simulink model "PSOmodel"  (R2023a)
settings: Solver=FixedStepAuto  StartTime=0.0  StopTime=19431  FixedStep=1  RelTol=1e-3
undefined symbols (not defined in the file): G, PSO

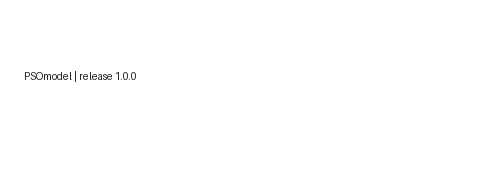
[thumbnail: Simulink's stored preview of the top-level diagram]
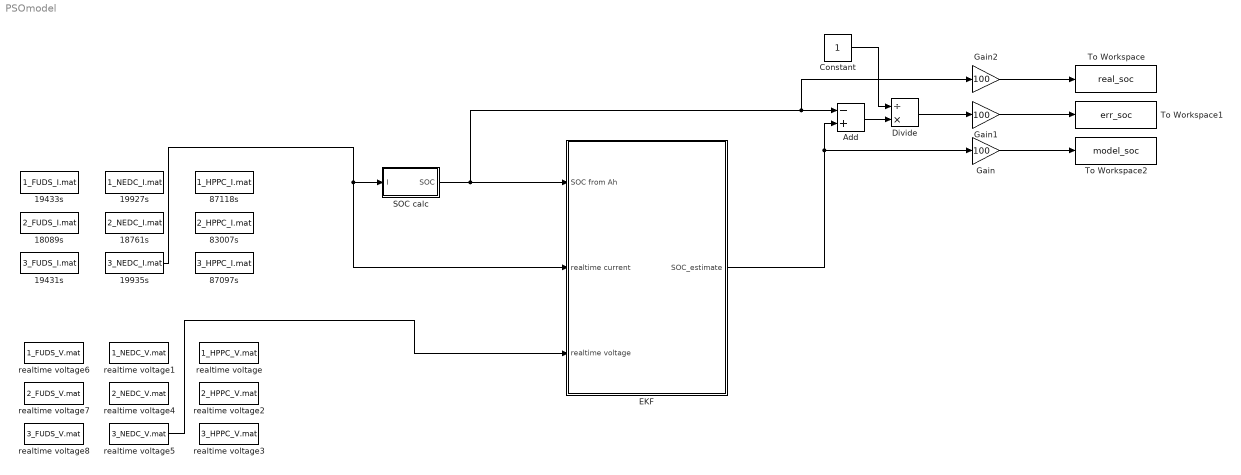
== system PSOmodel ==
  18089s : FromFile  FileName=2_FUDS_I.mat  SampleTime=0
  18761s : FromFile  FileName=2_NEDC_I.mat  SampleTime=0
  19431s : FromFile  FileName=3_FUDS_I.mat  SampleTime=0
  19433s : FromFile  FileName=1_FUDS_I.mat  SampleTime=0
  19927s : FromFile  FileName=1_NEDC_I.mat  SampleTime=0
  19935s : FromFile  FileName=3_NEDC_I.mat  SampleTime=0
  83007s : FromFile  FileName=2_HPPC_I.mat  SampleTime=0
  87097s : FromFile  FileName=3_HPPC_I.mat  SampleTime=0
  87118s : FromFile  FileName=1_HPPC_I.mat  SampleTime=0
  Add : Sum  Inputs=-+
  Constant : Constant
  Divide : Product  Inputs=/*
  EKF : Subsystem
  Gain : Gain  Gain=100
  Gain1 : Gain  Gain=100
  Gain2 : Gain  Gain=100
  SOC calc : Subsystem
  To Workspace : ToWorkspace  VariableName=real_soc  SaveFormat=Timeseries  SampleTime=-1
  To Workspace1 : ToWorkspace  VariableName=err_soc  SaveFormat=Timeseries  SampleTime=-1
  To Workspace2 : ToWorkspace  VariableName=model_soc  SaveFormat=Timeseries  SampleTime=-1
  realtime voltage : FromFile  FileName=1_HPPC_V.mat  SampleTime=0
  realtime voltage1 : FromFile  FileName=1_NEDC_V.mat  SampleTime=0
  realtime voltage2 : FromFile  FileName=2_HPPC_V.mat  SampleTime=0
  realtime voltage3 : FromFile  FileName=3_HPPC_V.mat  SampleTime=0
  realtime voltage4 : FromFile  FileName=2_NEDC_V.mat  SampleTime=0
  realtime voltage5 : FromFile  FileName=3_NEDC_V.mat  SampleTime=0
  realtime voltage6 : FromFile  FileName=1_FUDS_V.mat  SampleTime=0
  realtime voltage7 : FromFile  FileName=2_FUDS_V.mat  SampleTime=0
  realtime voltage8 : FromFile  FileName=3_FUDS_V.mat  SampleTime=0
  wires:
  19935s/1 -> EKF/2(realtime current), SOC calc/1(I)
  EKF/1(SOC_estimate) -> Gain/1, Add/2
  Add/1 -> Divide/2
  realtime voltage5/1 -> EKF/3("realtime voltage ")
  Divide/1 -> Gain1/1
  Gain/1 -> To Workspace2/1
  Constant/1 -> Divide/1
  Gain2/1 -> To Workspace/1
  Gain1/1 -> To Workspace1/1
  SOC calc/1(SOC) -> Gain2/1, Add/1, EKF/1(SOC from Ah)

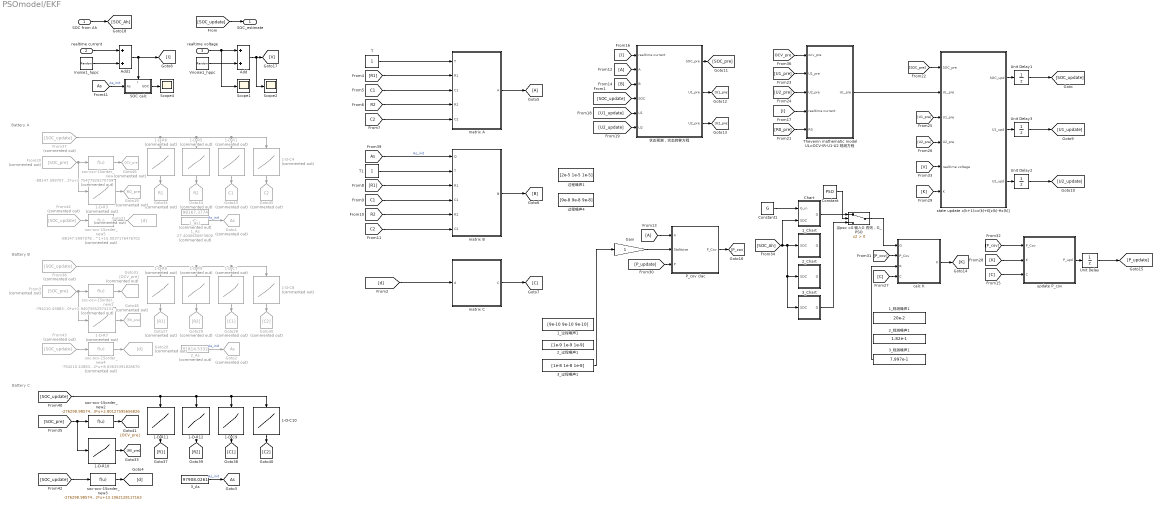
== system PSOmodel/EKF ==
  note: Battery C
  note: Battery B
  note: Battery A
  SOC from Ah : Inport
  realtime current : Inport  Port=2
  "realtime voltage " : Inport  Port=3
  1-D-C10 : Lookup_n-D  NumberOfTableDimensions=1  BreakpointsForDimension1=[2.9109E-07, 0.034704903, 0.080678392, 0.126651918, 0.172626069, 0.218599963, 0.264561539, 0.310535727, 0.35649723, 0.402458916, 0.448432994, 0.494395195, 0.540356772, 0.586318863, 0.632281101, 0.678243265, 0.724205797, 0.770168256, 0.81613042, 0.862092732, 0.908054492, 0.954027467]  Table=[2196.493417, 6254.414395, 10027.09575, 11640.94595, 15150.56735, 14939.39571, 22277.23726, 21788.57636, 21198.25628, 16155.2285, 17423.71863, 20324.46195, 14880.37747, 17370.84513, 17908.76661, 37791.77026, 30450.72328, 20196.6933, 17282.88891, 15011.20802, 15927.09163, 25703.81768]  InternalRulePriority=Speed  RndMeth=Simplest
  1-D-C4 : Lookup_n-D  Commented=on  NumberOfTableDimensions=1  BreakpointsForDimension1=[-1.87350000000000e-16 0.0372369600000000 0.0830859250000000 0.128934580000000 0.174779663000000 0.220625308000000 0.266470959000000 0.312315714000000 0.358160890000000 0.404006225000000 0.449851236000000 0.495695831000000 0.541540865000000 0.587386376000000 0.633231553000000 0.679076361000000 0.724921708000000 0.770765746000000 0.816610252000000 0.862454330000000 0.908300370000000 0.954150372000000]  Table=[128354.582000000 465098.236000000 494756.285300000 743304.727400000 722463.651900000 811208.927300000 406248.240800000 454089.078800000 480121.157400000 703814.335700000 645290.670500000 845206.089900000 863339.383500000 831786.696500000 413452.541700000 382645.914900000 796268.796700000 831394.125000000 798423.035300000 722500.010700000 1812473.80600000 1386271.68100000]  InternalRulePriority=Speed  RndMeth=Simplest
  1-D-C7 : Lookup_n-D  Commented=on  NumberOfTableDimensions=1  BreakpointsForDimension1=[-7.8419E-08, 0.019714291, 0.068728061, 0.117742026, 0.166756071, 0.21576937, 0.264783571, 0.313798204, 0.362812366, 0.411826096, 0.460839905, 0.50985442, 0.55886819, 0.60788247, 0.656896828, 0.705911421, 0.754926406, 0.803941313, 0.852956063, 0.901970617, 0.950985446]  Table=[225214.1434, 187025.2766, 296294.3583, 325129.1549, 382794.7295, 371710.2995, 353976.6676, 381282.3938, 488296.3231, 462238.5316, 712185.7898, 891276.2929, 786232.5864, 455006.0004, 322811.3497, 309379.8901, 321116.448, 741388.8307, 942394.5955, 1060535.922, 1063695.943]  InternalRulePriority=Speed  RndMeth=Simplest
  1-D-C8 : Lookup_n-D  Commented=on  NumberOfTableDimensions=1  BreakpointsForDimension1=[-7.8419E-08, 0.019714291, 0.068728061, 0.117742026, 0.166756071, 0.21576937, 0.264783571, 0.313798204, 0.362812366, 0.411826096, 0.460839905, 0.50985442, 0.55886819, 0.60788247, 0.656896828, 0.705911421, 0.754926406, 0.803941313, 0.852956063, 0.901970617, 0.950985446]  Table=[1671.127633, 1673.968389, 4565.243665, 6209.535618, 11242.6131, 9787.657058, 11449.06044, 14014.79555, 15699.36024, 13663.69917, 14717.09328, 14685.37445, 16462.66037, 11898.52641, 12704.67604, 16178.70649, 18177.54925, 20734.64693, 17610.56739, 15941.06135, 15784.62672]  InternalRulePriority=Speed  RndMeth=Simplest
  1-D-C9 : Lookup_n-D  NumberOfTableDimensions=1  BreakpointsForDimension1=[2.9109E-07, 0.034704903, 0.080678392, 0.126651918, 0.172626069, 0.218599963, 0.264561539, 0.310535727, 0.35649723, 0.402458916, 0.448432994, 0.494395195, 0.540356772, 0.586318863, 0.632281101, 0.678243265, 0.724205797, 0.770168256, 0.81613042, 0.862092732, 0.908054492, 0.954027467]  Table=[148211.7874, 379943.691, 507178.8648, 540877.9099, 565031.5977, 599113.5276, 468851.5567, 439228.3613, 564632.19, 525250.0917, 713932.6032, 938377.816, 623343.6413, 597265.7355, 374444.1491, 318686.1875, 638311.9656, 790877.9592, 883896.1639, 825362.4483, 795349.2136, 1510862.771]  InternalRulePriority=Speed  RndMeth=Simplest
  1-D-R1 : Lookup_n-D  Commented=on  NumberOfTableDimensions=1  BreakpointsForDimension1=[-1.87350000000000e-16 0.0372369600000000 0.0830859250000000 0.128934580000000 0.174779663000000 0.220625308000000 0.266470959000000 0.312315714000000 0.358160890000000 0.404006225000000 0.449851236000000 0.495695831000000 0.541540865000000 0.587386376000000 0.633231553000000 0.679076361000000 0.724921708000000 0.770765746000000 0.816610252000000 0.862454330000000 0.908300370000000 0.954150372000000]  Table=[0.00810316000000000 0.00251698500000000 0.00186214400000000 0.00178860800000000 0.00152974100000000 0.00147679700000000 0.00190128400000000 0.00201018500000000 0.00174515000000000 0.00143752800000000 0.00133514600000000 0.00126586900000000 0.00125399700000000 0.00138251100000000 0.00279094200000000 0.00218289100000000 0.00138689300000000 0.00122421400000000 0.00113694900000000 0.00107976200000000 0.000788270000000000 0.000893057000000000]  InternalRulePriority=Speed  RndMeth=Simplest
  1-D-R10 : Lookup_n-D  NumberOfTableDimensions=1  BreakpointsForDimension1=[2.9109E-07, 0.034704903, 0.080678392, 0.126651918, 0.172626069, 0.218599963, 0.264561539, 0.310535727, 0.35649723, 0.402458916, 0.448432994, 0.494395195, 0.540356772, 0.586318863, 0.632281101, 0.678243265, 0.724205797, 0.770168256, 0.81613042, 0.862092732, 0.908054492, 0.954027467]  Table=[0.002528647, 0.001936736, 0.001933092, 0.002009272, 0.001857034, 0.001932965, 0.001937093, 0.001860779, 0.001865146, 0.001940916, 0.001785007, 0.001860795, 0.001784893, 0.001792897, 0.001860957, 0.001860919, 0.001788901, 0.0017849, 0.001708766, 0.001708843, 0.001636824, 0.001636826]  InternalRulePriority=Speed  RndMeth=Simplest
  1-D-R11 : Lookup_n-D  NumberOfTableDimensions=1  BreakpointsForDimension1=[2.9109E-07, 0.034704903, 0.080678392, 0.126651918, 0.172626069, 0.218599963, 0.264561539, 0.310535727, 0.35649723, 0.402458916, 0.448432994, 0.494395195, 0.540356772, 0.586318863, 0.632281101, 0.678243265, 0.724205797, 0.770168256, 0.81613042, 0.862092732, 0.908054492, 0.954027467]  Table=[0.007426917, 0.002725754, 0.002056684, 0.002051955, 0.001788462, 0.001933155, 0.002069724, 0.00225684, 0.001884435, 0.0016594, 0.001488249, 0.001395496, 0.001419538, 0.001566898, 0.002844649, 0.002781912, 0.001682693, 0.00138196, 0.001233272, 0.001177427, 0.001101257, 0.000924041]  InternalRulePriority=Speed  RndMeth=Simplest
  1-D-R12 : Lookup_n-D  NumberOfTableDimensions=1  BreakpointsForDimension1=[2.9109E-07, 0.034704903, 0.080678392, 0.126651918, 0.172626069, 0.218599963, 0.264561539, 0.310535727, 0.35649723, 0.402458916, 0.448432994, 0.494395195, 0.540356772, 0.586318863, 0.632281101, 0.678243265, 0.724205797, 0.770168256, 0.81613042, 0.862092732, 0.908054492, 0.954027467]  Table=[0.012678994, 0.006218342, 0.004585322, 0.003481865, 0.003212414, 0.002922909, 0.002535113, 0.002663285, 0.002728817, 0.002644002, 0.002455207, 0.0022745, 0.002186381, 0.002057863, 0.001998786, 0.002105164, 0.002862673, 0.002808045, 0.002531815, 0.002274687, 0.00198128, 0.001756841]  InternalRulePriority=Speed  RndMeth=Simplest
  1-D-R3 : Lookup_n-D  Commented=on  NumberOfTableDimensions=1  BreakpointsForDimension1=[-1.87350000000000e-16 0.0372369600000000 0.0830859250000000 0.128934580000000 0.174779663000000 0.220625308000000 0.266470959000000 0.312315714000000 0.358160890000000 0.404006225000000 0.449851236000000 0.495695831000000 0.541540865000000 0.587386376000000 0.633231553000000 0.679076361000000 0.724921708000000 0.770765746000000 0.816610252000000 0.862454330000000 0.908300370000000 0.954150372000000]  Table=[0.00237719800000000 0.00193720900000000 0.00163261400000000 0.00164061700000000 0.00163282300000000 0.00148875000000000 0.00148875000000000 0.00164061700000000 0.00164082700000000 0.00148892900000000 0.00148912000000000 0.00148875000000000 0.00148875000000000 0.00148875000000000 0.00148875000000000 0.00148856000000000 0.00148892900000000 0.00134450600000000 0.00134467800000000 0.00148856000000000 0.00164082700000000 0.00148856000000000]  InternalRulePriority=Speed  RndMeth=Simplest
  1-D-R5 : Lookup_n-D  Commented=on  NumberOfTableDimensions=1  BreakpointsForDimension1=[-1.87350000000000e-16 0.0372369600000000 0.0830859250000000 0.128934580000000 0.174779663000000 0.220625308000000 0.266470959000000 0.312315714000000 0.358160890000000 0.404006225000000 0.449851236000000 0.495695831000000 0.541540865000000 0.587386376000000 0.633231553000000 0.679076361000000 0.724921708000000 0.770765746000000 0.816610252000000 0.862454330000000 0.908300370000000 0.954150372000000]  Table=[0.00810316000000000 0.00251698500000000 0.00186214400000000 0.00178860800000000 0.00152974100000000 0.00147679700000000 0.00190128400000000 0.00201018500000000 0.00174515000000000 0.00143752800000000 0.00133514600000000 0.00126586900000000 0.00125399700000000 0.00138251100000000 0.00279094200000000 0.00218289100000000 0.00138689300000000 0.00122421400000000 0.00113694900000000 0.00107976200000000 0.000788270000000000 0.000893057000000000]  InternalRulePriority=Speed  RndMeth=Simplest
  1-D-R6 : Lookup_n-D  Commented=on  NumberOfTableDimensions=1  BreakpointsForDimension1=[-1.87350000000000e-16 0.0372369600000000 0.0830859250000000 0.128934580000000 0.174779663000000 0.220625308000000 0.266470959000000 0.312315714000000 0.358160890000000 0.404006225000000 0.449851236000000 0.495695831000000 0.541540865000000 0.587386376000000 0.633231553000000 0.679076361000000 0.724921708000000 0.770765746000000 0.816610252000000 0.862454330000000 0.908300370000000 0.954150372000000]  Table=[0.00853642300000000 0.00464516200000000 0.00372978500000000 0.00280459900000000 0.00271064400000000 0.00238071300000000 0.00215293400000000 0.00228803900000000 0.00239974300000000 0.00228676500000000 0.00209879800000000 0.00194772300000000 0.00181591800000000 0.00170293300000000 0.00173486000000000 0.00212977600000000 0.00261638200000000 0.00242766200000000 0.00219563000000000 0.00194553200000000 0.00171752800000000 0.00157829700000000]  InternalRulePriority=Speed  RndMeth=Simplest
  1-D-R7 : Lookup_n-D  Commented=on  NumberOfTableDimensions=1  BreakpointsForDimension1=[-7.8419E-08, 0.019714291, 0.068728061, 0.117742026, 0.166756071, 0.21576937, 0.264783571, 0.313798204, 0.362812366, 0.411826096, 0.460839905, 0.50985442, 0.55886819, 0.60788247, 0.656896828, 0.705911421, 0.754926406, 0.803941313, 0.852956063, 0.901970617, 0.950985446]  Table=[0.005142418, 0.004920407, 0.004844512, 0.004848168, 0.00477236, 0.004844207, 0.004916611, 0.004768351, 0.004768354, 0.004767743, 0.004920582, 0.00484046, 0.004695644, 0.004619808, 0.004547664, 0.004543704, 0.004467293, 0.004547664, 0.004547368, 0.004399462, 0.004246964]  InternalRulePriority=Speed  RndMeth=Simplest
  1-D-R8 : Lookup_n-D  Commented=on  NumberOfTableDimensions=1  BreakpointsForDimension1=[-7.8419E-08, 0.019714291, 0.068728061, 0.117742026, 0.166756071, 0.21576937, 0.264783571, 0.313798204, 0.362812366, 0.411826096, 0.460839905, 0.50985442, 0.55886819, 0.60788247, 0.656896828, 0.705911421, 0.754926406, 0.803941313, 0.852956063, 0.901970617, 0.950985446]  Table=[0.00461437, 0.004542772, 0.002927848, 0.002489007, 0.00261231, 0.002854022, 0.002839665, 0.002705643, 0.002322517, 0.001930102, 0.001569536, 0.001434529, 0.001559029, 0.002338951, 0.003742684, 0.00311492, 0.00238201, 0.001540864, 0.001263662, 0.001122294, 0.001006783]  InternalRulePriority=Speed  RndMeth=Simplest
  1-D-R9 : Lookup_n-D  Commented=on  NumberOfTableDimensions=1  BreakpointsForDimension1=[-7.8419E-08, 0.019714291, 0.068728061, 0.117742026, 0.166756071, 0.21576937, 0.264783571, 0.313798204, 0.362812366, 0.411826096, 0.460839905, 0.50985442, 0.55886819, 0.60788247, 0.656896828, 0.705911421, 0.754926406, 0.803941313, 0.852956063, 0.901970617, 0.950985446]  Table=[0.022805443, 0.021704309, 0.009347226, 0.005943316, 0.004810936, 0.004550218, 0.004093036, 0.003809411, 0.003763955, 0.003626777, 0.003515244, 0.003368593, 0.002718876, 0.003041587, 0.003017746, 0.002947958, 0.003081328, 0.00338066, 0.003232809, 0.003004131, 0.002690434]  InternalRulePriority=Speed  RndMeth=Simplest
  1_As : Constant  Commented=on  Value=27.40406506*3600
  1_As1 : Constant  Commented=on  Value=98167.3774
  1_Chart : Stateflow chart  TreatAsAtomicUnit=on
  1_观测噪声1 : Constant  Value=20e-2
  1_过程噪声1 : Constant  Value=[9e-10 9e-10 9e-10]
  2_As : Constant  Commented=on  Value=91814.5332
  2_Chart : Stateflow chart  TreatAsAtomicUnit=on
  2_观测噪声1 : Constant  Value=1.82e-1
  2_过程噪声1 : Constant  Value=[1e-9 1e-9 1e-9]
  3_As : Constant  Value=97908.0261
  3_Chart : Stateflow chart  TreatAsAtomicUnit=on
  3_观测噪声1 : Constant  Value=7.997e-1  VectorParams1D=off
  3_过程噪声1 : Constant  Value=[1e-8 1e-8 1e-8]
  Add : Sum
  Add1 : Sum
  Chart : Stateflow chart  TreatAsAtomicUnit=on
      settings: PortSchema="{\"entries\":[{\"content\":{\"sides\":[{\"content\":{\"connectorIds\":[\"In2\",\"In1\"]},\"type\":\"ConnectorPlacement.EquallySpacedRectSide\",\"uuid\":\"e7012a5c-4e88-428d-83d6-0abb774271f4\"},{\"content\":{\"connectorIds\":[\"Out1\"],\"side\":\"RIGHT\"},\"type\":\"ConnectorPlacement.EquallySpacedRectSide\",\"uuid\":\"a64351c2-cb69-49cc-89e3-a743088e35f9\"},{\"content\":{\"side\":\"TOP\"},\"type\":\"ConnectorPlacement.EquallySpacedRectSide\",\"uuid\":\"04fad1cd-d4dd-41b0-a559-7d397359cb8e\"}]},\"type\":\"ConnectorPlacement.EquallySpacedConnector\",\"uuid\":\"62b6021a-e1f5-4386-ac4f-7a5c61b690a4\"}],\"packageUris\":[\"http://schema.mathworks.com/mf0/Connector/R2020b\"],\"version\":\"1.0\"}"
  Constant : Constant  Value=PSO
  Constant1 : Constant  Value=G
  From12 : From
  From13 : From
  From20 : From  Commented=on  GotoTag=SOC_pre
  From3 : From  Commented=on  GotoTag=SOC_pre
  From{37..38,43..44} (4 alike) : From  Commented=on  GotoTag=SOC_update
  Gain : Gain
  Goto1 : Goto  Commented=on  GotoTag=As  TagVisibility=global
  Goto19 : Goto  Commented=on  GotoTag=R0_pre  TagVisibility=global
  Goto2 : Goto  Commented=on  GotoTag=As  TagVisibility=global
  Goto20 : Goto  Commented=on  GotoTag=d
  Goto21 : Goto  Commented=on  GotoTag=d
  Goto27 : Goto  Commented=on  GotoTag=R1
  Goto28 : Goto  Commented=on  GotoTag=C1
  Goto29 : Goto  Commented=on  GotoTag=R2
  Goto30 : Goto  Commented=on  GotoTag=C2
  Goto31 : Goto  Commented=on  GotoTag=OCV_pre
  Goto34 : Goto  Commented=on  GotoTag=R1  TagVisibility=global
  Goto43 : Goto  Commented=on  GotoTag=C1  TagVisibility=global
  Goto44 : Goto  Commented=on  GotoTag=R2  TagVisibility=global
  Goto45 : Goto  Commented=on  GotoTag=C2  TagVisibility=global
  Goto46 : Goto  Commented=on  GotoTag=OCV_pre  TagVisibility=global
  Goto48 : Goto  Commented=on  GotoTag=R0_pre
  Goto5 : Goto
  Inoise1_hppc : RandomNumber  Mean=0.01  Variance=1e-7  SampleTime=0
  P_cov clac : MATLAB Function  TreatAsAtomicUnit=on
  SOC calc : Subsystem
      settings: PortSchema="{\"entries\":[{\"content\":{\"sides\":[{\"content\":{\"connectorIds\":[\"In1\"]},\"type\":\"ConnectorPlacement.EquallySpacedRectSide\",\"uuid\":\"9a15624f-070f-46ab-b122-3cccf513f6e5\"},{\"content\":{\"connectorIds\":[\"Out1\"],\"side\":\"RIGHT\"},\"type\":\"ConnectorPlacement.EquallySpacedRectSide\",\"uuid\":\"7075dd8f-f637-4b75-9ab6-2a45eadbfae6\"},{\"content\":{\"connectorIds\":[\"In2\"],\"side\":\"TOP\"},\"type\":\"ConnectorPlacement.EquallySpacedRectSide\",\"uuid\":\"a2ff706a-1abd-4808-a923-af34f3449a3c\"}]},\"type\":\"ConnectorPlacement.EquallySpacedConnector\",\"uuid\":\"893fac7f-2ce4-44cf-9782-68cb5d4c65ac\"}],\"packageUris\":[\"http://schema.mathworks.com/mf0/Connector/R2020b\"],\"version\":\"1.0\"}"
  Scope1 : Scope
  Scope2 : Scope
  Scope4 : Scope
  T : Constant
  T1 : Constant
  Thevenin mathematic model UL=OCV-IR-U1-U2 观测方程 : Subsystem  TreatAsAtomicUnit=on
  Unit Delay : UnitDelay  InitialCondition=[0.01,0,0,0,0.01,0,0,0,0.01]  SampleTime=-1  HasFrameUpgradeWarning=on
  Unit Delay1 : UnitDelay  InitialCondition=0.95  HasFrameUpgradeWarning=on
  Unit Delay2 : UnitDelay  InitialCondition=0.5  HasFrameUpgradeWarning=on
  Unit Delay3 : UnitDelay  InitialCondition=0.5  HasFrameUpgradeWarning=on
  Vnoise1_hppc : RandomNumber  Mean=0.001  Variance=1e-9  SampleTime=0
  calc K : MATLAB Function  TreatAsAtomicUnit=on
  matrix A : Subsystem  TreatAsAtomicUnit=on
  matrix B : Subsystem  TreatAsAtomicUnit=on
  matrix C : Subsystem  TreatAsAtomicUnit=on
  soc-ocv-15order_new : Fcn  Commented=on  Expr=-88147.5997078394*u^15+790326.983827153*u^14-3193562.76566965*u^13+7683743.41545882*u^12-12242299.9696135*u^11+13582405.847664*u^10-10735891.8510933*u^9+6074345.19664904*u^8-2430691.37715694*u^7+664003.897026294*u^6-113520.233149201*u^5+8942.36593610576*u^4+511.723044470873*u^3-179.974721169225*u^2+15.0037176476702*u+2.75477929270709
  soc-ocv-15order_new1 : Fcn  Commented=on  Expr=-794210.438834610*u^15+5987745.61568300*u^14-20439836.7898101*u^13+41772168.8258101*u^12-56921777.5690841*u^11+54490938.0492044*u^10-37586563.2858994*u^9+18834958.2927790*u^8-6814558.32935900*u^7+1740625.65248685*u^6-299189.844437199*u^5+31109.3414812153*u^4-1360.69378520401*u^3-57.0272510664786*u^2+8.63635391828670*u+2.94075652974131
  soc-ocv-15order_new2 : Fcn  Expr=-276298.985749310*u^15+2079100.19510310*u^14-7146107.09932892*u^13+14857923.9617195*u^12-20833240.2231729*u^11+20756759.1140984*u^10-15054210.4175051*u^9+7991543.21304879*u^8-3070959.05248522*u^7+827625.466792177*u^6-145769.880033493*u^5+13780.6338711194*u^4-19.7560716602156*u^3-139.705484335419*u^2+13.1062128117163*u+2.80127595656826
  soc-ocv-15order_new3 : Fcn  Expr=-276298.985749310*15*u^14+2079100.19510310*14*u^13-7146107.09932892*13*u^12+14857923.9617195*12*u^11-20833240.2231729*11*u^10+20756759.1140984*10*u^9-15054210.4175051*9*u^8+7991543.21304879*8*u^7-3070959.05248522*7*u^6+827625.466792177*6*u^5-145769.880033493*5*u^4+13780.6338711194*4*u^3-19.7560716602156*3*u^2-139.705484335419*2*u+13.1062128117163
  soc-ocv-15order_new4 : Fcn  Commented=on  Expr=-794210.438834610*15*u^14+5987745.61568300*14*u^13-20439836.7898101*13*u^12+41772168.8258101*12*u^11-56921777.5690841*11*u^10+54490938.0492044*10*u^9-37586563.2858994*9*u^8+18834958.2927790*8*u^7-6814558.32935900*7*u^6+1740625.65248685*6*u^5-299189.844437199*5*u^4+31109.3414812153*4*u^3-1360.69378520401*3*u^2-57.0272510664786*2*u+8.63635391828670
  soc-ocv-15order_new5 : Fcn  Commented=on  Expr=-88147.5997078394*15*u^14+790326.983827153*14*u^13-3193562.76566965*13*u^12+7683743.41545882*12*u^11-12242299.9696135*11*u^10+13582405.847664*10*u^9-10735891.8510933*9*u^8+6074345.19664904*8*u^7-2430691.37715694*7*u^6+664003.897026294*6*u^5-113520.233149201*5*u^4+8942.36593610576*4*u^3+511.723044470873*3*u^2-179.974721169225*2*u^1+15.0037176476702
  state update x(k+1)=x(k)+K[z(k)-Hx(k)] : Subsystem
  update P_cov : MATLAB Function  TreatAsAtomicUnit=on
  当pso >0 输入G 否则，G_PSO : Switch  Criteria=u2 > Threshold  SaturateOnIntegerOverflow=off  InputSameDT=off
  状态预测，状态转移方程 : Subsystem
  过程噪声1 : Constant  Value=[2e-5 1e-5 1e-5]
  过程噪声4 : Constant  Value=[9e-8 9e-8 9e-8]
  SOC_estimate : Outport
  tag scope: As=global
  wires:
  [As] -> matrix B/1(Q)  "As_init"
  [C] -> update P_cov/3(C)
  [U2_pre] -> Thevenin mathematic model UL=OCV-IR-U1-U2 观测方程/3(U2_pre)
  [OCV_pre] -> Thevenin mathematic model UL=OCV-IR-U1-U2 观测方程/1(ocv_pre)
  [U1_pre] -> Thevenin mathematic model UL=OCV-IR-U1-U2 观测方程/2(U1_pre)
  state update x(k+1)=x(k)+K[z(k)-Hx(k)]/2(U1_upd) -> Unit Delay3/1
  state update x(k+1)=x(k)+K[z(k)-Hx(k)]/3(U2_upd) -> Unit Delay2/1
  T/1 -> matrix A/1(T)
  state update x(k+1)=x(k)+K[z(k)-Hx(k)]/1(SOC_upd) -> Unit Delay1/1
  Thevenin mathematic model UL=OCV-IR-U1-U2 观测方程/1(UL_pre) -> state update x(k+1)=x(k)+K[z(k)-Hx(k)]/2(UL_pre)
  update P_cov/1(P_upd) -> Unit Delay/1
  Gain/1 -> P_cov clac/2(StaNoise)
  3_Chart/1(G) -> 当pso >0 输入G 否则，G_PSO/3
  [SOC_update] -> SOC_estimate/1
  T1/1 -> matrix B/2(T)
  [SOC_update] -> 状态预测，状态转移方程/4(SOC)
  [d] -> matrix C/1(d)
  [R1] -> matrix A/2(R1)
  [C1] -> matrix A/3(C1)
  [R2] -> matrix A/4(R2)
  [C2] -> matrix A/5(C2)
  [R1] -> matrix B/3(R1)
  [C1] -> matrix B/4(C1)
  [R2] -> matrix B/5(R2)
  [C2] -> matrix B/6(C2)
  matrix A/1(A) -> Goto5/1
  matrix B/1(B) -> [B]
  From12/1 -> 状态预测，状态转移方程/2(A)
  From13/1 -> P_cov clac/1(A)
  [B] -> 状态预测，状态转移方程/3(B)
  matrix C/1(C) -> [C]
  realtime current/1 -> Add1/1
  [I] -> 状态预测，状态转移方程/1(realtime current)
  [I] -> Thevenin mathematic model UL=OCV-IR-U1-U2 观测方程/4(realtime current)
  Unit Delay3/1 -> [U1_update]
  Unit Delay2/1 -> [U2_update]
  [U1_update] -> 状态预测，状态转移方程/5(U1)
  [U2_update] -> 状态预测，状态转移方程/6(U2)
  [SOC_pre] -> state update x(k+1)=x(k)+K[z(k)-Hx(k)]/1(SOC_pre)
  状态预测，状态转移方程/2(U1_pre) -> [U1_pre]
  状态预测，状态转移方程/3(U2_pre) -> [U2_pre]
  [U1_pre] -> state update x(k+1)=x(k)+K[z(k)-Hx(k)]/3(U1_pre)
  [U2_pre] -> state update x(k+1)=x(k)+K[z(k)-Hx(k)]/4(U2_pre)
  [C] -> calc K/4(C)
  calc K/1(K) -> [K]
  [K] -> update P_cov/2(K)
  [K] -> state update x(k+1)=x(k)+K[z(k)-Hx(k)]/6(K)
  Unit Delay/1 -> [P_update]
  [P_update] -> P_cov clac/3(P)
  P_cov clac/1(P_Cov) -> [P_cov]
  [P_cov] -> calc K/2(P_Cov)
  [P_cov] -> update P_cov/1(P_Cov)
  [V] -> state update x(k+1)=x(k)+K[z(k)-Hx(k)]/5(realtime voltage)
  SOC from Ah/1 -> [SOC_Ah]
  [SOC_Ah] -> Chart/1(SOC), 3_Chart/1(SOC), 2_Chart/1(SOC), 1_Chart/1(SOC)
  [R0_pre] -> Thevenin mathematic model UL=OCV-IR-U1-U2 观测方程/5(R0)
  Inoise1_hppc/1 -> Add1/2
  Add1/1 -> SOC calc/2(I), [I]
  Vnoise1_hppc/1 -> Add/2
  Add/1 -> Scope2/1, [V]
  "realtime voltage "/1 -> Scope1/1, Add/1
  状态预测，状态转移方程/1(SOC_pre) -> [SOC_pre]
  SOC calc/1(SOC) -> Scope4/1
  Unit Delay1/1 -> [SOC_update]
  soc-ocv-15order_new2/1 -> [OCV_pre]
  1-D-C4/1 -> Goto45/1
  1-D-R12/1 -> [R2]
  1-D-R11/1 -> [R1]
  From37/1 -> 1-D-R6/1, 1-D-R5/1, 1-D-C4/1, 1-D-R1/1
  1-D-C10/1 -> [C2]
  1-D-R9/1 -> Goto29/1
  1-D-R10/1 -> [R0_pre]
  From38/1 -> 1-D-C8/1, 1-D-C7/1, 1-D-R9/1, 1-D-R8/1
  [SOC_update] -> 1-D-C10/1, 1-D-C9/1, 1-D-R12/1, 1-D-R11/1
  1-D-R8/1 -> Goto27/1
  1-D-R5/1 -> Goto44/1
  1-D-R3/1 -> Goto19/1
  1-D-R7/1 -> Goto48/1
  soc-ocv-15order_new1/1 -> Goto31/1
  1-D-C8/1 -> Goto30/1
  1-D-C7/1 -> Goto28/1
  1-D-R1/1 -> Goto43/1
  1-D-R6/1 -> Goto34/1
  soc-ocv-15order_new/1 -> Goto46/1
  1-D-C9/1 -> [C1]
  From20/1 -> 1-D-R3/1, soc-ocv-15order_new/1
  From3/1 -> soc-ocv-15order_new1/1, 1-D-R7/1
  [SOC_pre] -> 1-D-R10/1, soc-ocv-15order_new2/1
  [As] -> SOC calc/1(As)  "As_init"
  1_As/1 -> Goto1/1  "As_init"
  3_As/1 -> [As]  "As_init"
  2_As/1 -> Goto2/1  "As_init"
  [SOC_update] -> soc-ocv-15order_new3/1
  soc-ocv-15order_new3/1 -> [d]
  soc-ocv-15order_new4/1 -> Goto20/1
  From43/1 -> soc-ocv-15order_new4/1
  soc-ocv-15order_new5/1 -> Goto21/1
  From44/1 -> soc-ocv-15order_new5/1
  3_过程噪声1/1 -> Gain/1
  3_观测噪声1/1 -> calc K/3(R)
  当pso >0 输入G 否则，G_PSO/1 -> calc K/1(G)
  Constant/1 -> 当pso >0 输入G 否则，G_PSO/2
  Chart/1(G) -> 当pso >0 输入G 否则，G_PSO/1
  Constant1/1 -> Chart/2(G_in)

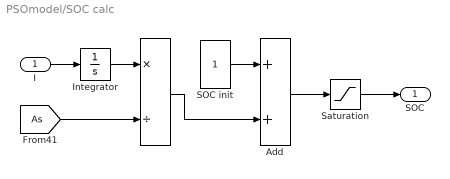
== system PSOmodel/SOC calc ==
  I : Inport
  "     " : Product  Inputs=*/
  Add : Sum
  Integrator : Integrator
  SOC init : Constant
  Saturation : Saturate  UpperLimit=1  LowerLimit=0
  SOC : Outport  VectorParamsAs1DForOutWhenUnconnected=off
  wires:
  [As] -> "     "/2
  Saturation/1 -> SOC/1
  SOC init/1 -> Add/1
  I/1 -> Integrator/1
  Integrator/1 -> "     "/1
  "     "/1 -> Add/2
  Add/1 -> Saturation/1

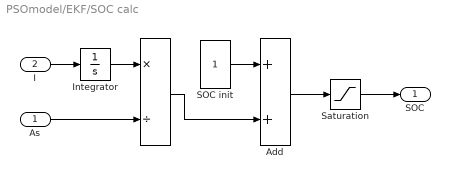
== system PSOmodel/EKF/SOC calc ==
  As : Inport
  I : Inport  Port=2
  "     " : Product  Inputs=*/
  Add : Sum
  Integrator : Integrator
  SOC init : Constant
  Saturation : Saturate  UpperLimit=1  LowerLimit=0
  SOC : Outport  VectorParamsAs1DForOutWhenUnconnected=off
  wires:
  As/1 -> "     "/2
  Saturation/1 -> SOC/1
  SOC init/1 -> Add/1
  I/1 -> Integrator/1
  Integrator/1 -> "     "/1
  "     "/1 -> Add/2
  Add/1 -> Saturation/1

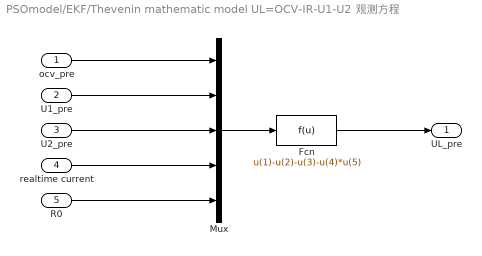
== system PSOmodel/EKF/Thevenin mathematic model UL=OCV-IR-U1-U2 观测方程 ==
  ocv_pre : Inport
  U1_pre : Inport  Port=2
  U2_pre : Inport  Port=3
  realtime current : Inport  Port=4
  R0 : Inport  Port=5
  Fcn : Fcn  Expr=u(1)-u(2)-u(3)-u(4)*u(5)
  Mux : Mux  Inputs=5
  UL_pre : Outport  VectorParamsAs1DForOutWhenUnconnected=off
  wires:
  Mux/1 -> Fcn/1
  ocv_pre/1 -> Mux/1
  U1_pre/1 -> Mux/2
  Fcn/1 -> UL_pre/1
  realtime current/1 -> Mux/4
  R0/1 -> Mux/5
  U2_pre/1 -> Mux/3

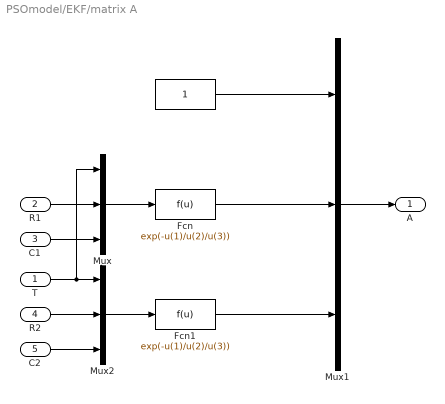
== system PSOmodel/EKF/matrix A ==
  T : Inport
  R1 : Inport  Port=2
  C1 : Inport  Port=3
  R2 : Inport  Port=4
  C2 : Inport  Port=5
  " " : Constant
  Fcn : Fcn  Expr=exp(-u(1)/u(2)/u(3))
  Fcn1 : Fcn  Expr=exp(-u(1)/u(2)/u(3))
  Mux : Mux  Inputs=3
  Mux1 : Mux  Inputs=3
  Mux2 : Mux  Inputs=3
  A : Outport  VectorParamsAs1DForOutWhenUnconnected=off
  wires:
  R1/1 -> Mux/2
  Fcn/1 -> Mux1/2
  T/1 -> Mux/1, Mux2/1
  C1/1 -> Mux/3
  Mux/1 -> Fcn/1
  " "/1 -> Mux1/1
  Mux1/1 -> A/1
  R2/1 -> Mux2/2
  C2/1 -> Mux2/3
  Mux2/1 -> Fcn1/1
  Fcn1/1 -> Mux1/3

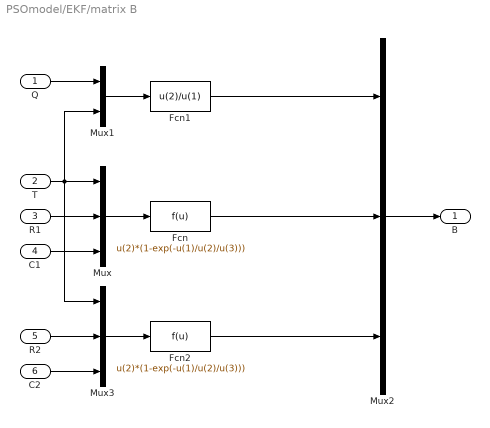
== system PSOmodel/EKF/matrix B ==
  Q : Inport
  T : Inport  Port=2
  R1 : Inport  Port=3
  C1 : Inport  Port=4
  R2 : Inport  Port=5
  C2 : Inport  Port=6
  Fcn : Fcn  Expr=u(2)*(1-exp(-u(1)/u(2)/u(3)))
  Fcn1 : Fcn  Expr=u(2)/u(1)
  Fcn2 : Fcn  Expr=u(2)*(1-exp(-u(1)/u(2)/u(3)))
  Mux : Mux  Inputs=3
  Mux1 : Mux  Inputs=2
  Mux2 : Mux  Inputs=3
  Mux3 : Mux  Inputs=3
  B : Outport  VectorParamsAs1DForOutWhenUnconnected=off
  wires:
  R1/1 -> Mux/2
  T/1 -> Mux3/1, Mux1/2, Mux/1
  C1/1 -> Mux/3
  Mux/1 -> Fcn/1
  Q/1 -> Mux1/1
  Mux1/1 -> Fcn1/1
  Fcn/1 -> Mux2/2
  Fcn1/1 -> Mux2/1
  Mux2/1 -> B/1
  R2/1 -> Mux3/2
  C2/1 -> Mux3/3
  Mux3/1 -> Fcn2/1
  Fcn2/1 -> Mux2/3

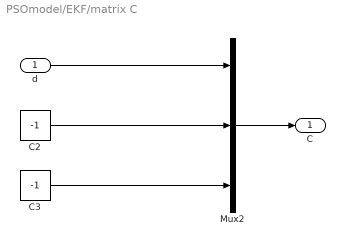
== system PSOmodel/EKF/matrix C ==
  d : Inport
  C2 : Constant  Value=-1
  C3 : Constant  Value=-1
  Mux2 : Mux  Inputs=3
  C : Outport  VectorParamsAs1DForOutWhenUnconnected=off
  wires:
  d/1 -> Mux2/1
  C2/1 -> Mux2/2
  Mux2/1 -> C/1
  C3/1 -> Mux2/3

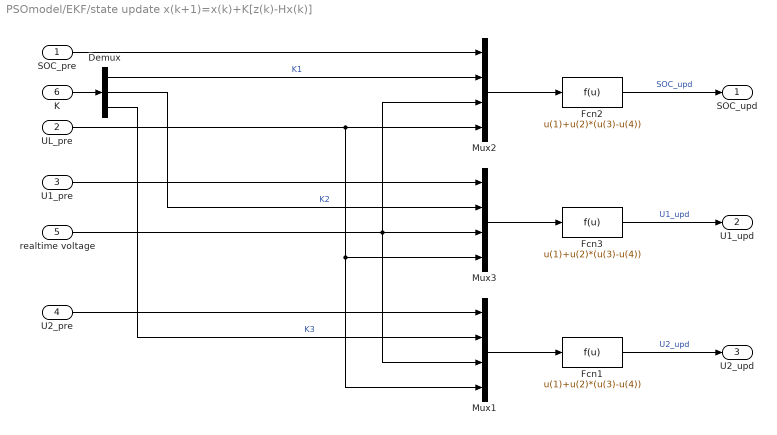
== system PSOmodel/EKF/state update x(k+1)=x(k)+K[z(k)-Hx(k)] ==
  SOC_pre : Inport
  UL_pre : Inport  Port=2
  U1_pre : Inport  Port=3
  U2_pre : Inport  Port=4
  realtime voltage : Inport  Port=5
  K : Inport  Port=6
  Demux : Demux  Outputs=3
  Fcn1 : Fcn  Expr=u(1)+u(2)*(u(3)-u(4))
  Fcn2 : Fcn  Expr=u(1)+u(2)*(u(3)-u(4))
  Fcn3 : Fcn  Expr=u(1)+u(2)*(u(3)-u(4))
  Mux1 : Mux
  Mux2 : Mux
  Mux3 : Mux
  SOC_upd : Outport  VectorParamsAs1DForOutWhenUnconnected=off
  U1_upd : Outport  Port=2  VectorParamsAs1DForOutWhenUnconnected=off
  U2_upd : Outport  Port=3  VectorParamsAs1DForOutWhenUnconnected=off
  wires:
  Fcn3/1 -> U1_upd/1  "U1_upd"
  Demux/1 -> Mux2/2  "K1"
  Demux/2 -> Mux3/2  "K2"
  Mux2/1 -> Fcn2/1
  Mux3/1 -> Fcn3/1
  K/1 -> Demux/1
  realtime voltage/1 -> Mux3/3, Mux2/3, Mux1/3
  UL_pre/1 -> Mux3/4, Mux1/4, Mux2/4
  U1_pre/1 -> Mux3/1
  SOC_pre/1 -> Mux2/1
  Fcn2/1 -> SOC_upd/1  "SOC_upd"
  Mux1/1 -> Fcn1/1
  Fcn1/1 -> U2_upd/1  "U2_upd"
  Demux/3 -> Mux1/2  "K3"
  U2_pre/1 -> Mux1/1

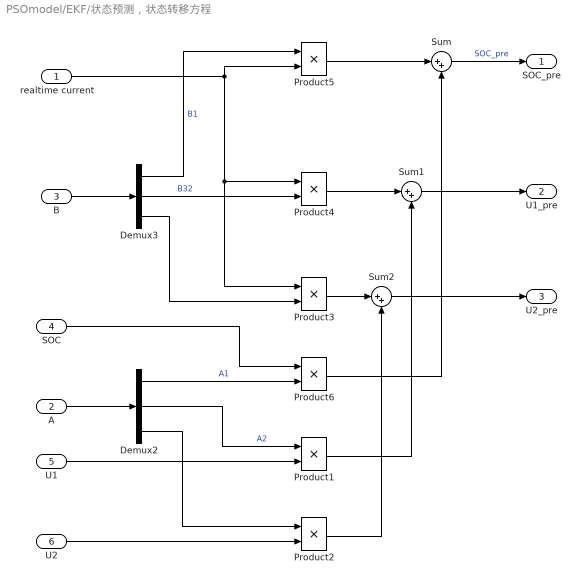
== system PSOmodel/EKF/状态预测，状态转移方程 ==
  realtime current : Inport
  A : Inport  Port=2
  B : Inport  Port=3
  SOC : Inport  Port=4
  U1 : Inport  Port=5
  U2 : Inport  Port=6
  Demux2 : Demux  Outputs=3
  Demux3 : Demux  Outputs=3
  Product{1..6} (6 alike) : Product
  Sum : Sum  Inputs=|++
  Sum1 : Sum  Inputs=|++
  Sum2 : Sum  Inputs=|++
  SOC_pre : Outport  VectorParamsAs1DForOutWhenUnconnected=off
  U1_pre : Outport  Port=2  VectorParamsAs1DForOutWhenUnconnected=off
  U2_pre : Outport  Port=3  VectorParamsAs1DForOutWhenUnconnected=off
  wires:
  Product5/1 -> Sum/1
  Demux2/2 -> Product1/1  "A2"
  A/1 -> Demux2/1
  Demux3/1 -> Product5/1  "B1"
  Product4/1 -> Sum1/1
  Sum1/1 -> U1_pre/1
  U1/1 -> Product1/2
  Product1/1 -> Sum1/2
  Sum/1 -> SOC_pre/1  "SOC_pre"
  B/1 -> Demux3/1
  Demux2/3 -> Product2/1
  U2/1 -> Product2/2
  Demux3/3 -> Product3/2
  realtime current/1 -> Product5/2, Product3/1, Product4/1
  Demux3/2 -> Product4/2  "B32"
  Product3/1 -> Sum2/1
  Sum2/1 -> U2_pre/1
  Product2/1 -> Sum2/2
  Demux2/1 -> Product6/2  "A1"
  SOC/1 -> Product6/1
  Product6/1 -> Sum/2

== stateflow chart PSOmodel/EKF/2_Chart ==
  (default) -> (junction 2)
  (junction 2) -> (junction 4) [order 1] : [SOC>0.6569&&SOC<0.7059]
  (junction 4) -> (junction 22) : {G=77.218/1000;}
  (junction 2) -> (junction 5) [order 2]
  (junction 5) -> (junction 6) [order 1] : [SOC>0.6079&&SOC<0.6569]
  (junction 6) -> (junction 28) : {G=35.657/1000;}
  (junction 5) -> (junction 18) [order 2]
  (junction 18) -> (junction 19) [order 1] : [SOC>0.5589&&SOC<0.6079]
  (junction 19) -> (junction 30) : {G=27.098/1000;}
  (junction 18) -> (junction 35) [order 2]
  (junction 35) -> (junction 36) [order 1] : [SOC>0.5099&&SOC<0.5589]
  (junction 36) -> (junction 40) : {G=27.161/1000;}
  (junction 35) -> (junction 43) [order 2]
  (junction 43) -> (junction 41) [order 1] : [SOC>0.4608&&SOC<0.5099]
  (junction 41) -> (junction 32) : {G=31.502/1000;}
  (junction 43) -> (junction 50) [order 2]
  (junction 50) -> (junction 47) [order 1] : [SOC>0.4118&&SOC<0.4608]
  (junction 47) -> (junction 56) : {G=36.53/1000;}
  (junction 50) -> (junction 48) [order 2]
  (junction 48) -> (junction 51) [order 1] : [SOC>0.3628&&SOC<0.4118]
  (junction 51) -> (junction 55) : {G=38.556/1000;}
  (junction 48) -> (junction 72) [order 2]
  (junction 72) -> (junction 70) [order 1] : [SOC>0.3138&&SOC<0.3628]
  (junction 70) -> (junction 44) : {G=38.822/1000;}
  (junction 72) -> (junction 59) [order 2]
  (junction 59) -> (junction 64) [order 1] : [SOC>0.2648&&SOC<0.3138]
  (junction 64) -> (junction 66) : {G=36.4/1000;}
  (junction 59) -> (junction 69) [order 2]
  (junction 69) -> (junction 63) [order 1] : [SOC>0.2158&&SOC<0.2648]
  (junction 63) -> (junction 60) : {G=31.972/1000;}
  (junction 69) -> (junction 80) [order 2]
  (junction 80) -> (junction 77) [order 1] : [SOC>0.1668&&SOC<0.2158]
  (junction 77) -> (junction 86) : {G=25.915/1000;}
  (junction 80) -> (junction 78) [order 2]
  (junction 78) -> (junction 81) [order 1] : [SOC>0.1177&&SOC<0.1668]
  (junction 81) -> (junction 85) : {G=22.037/1000;}
  (junction 78) -> (junction 102) [order 2]
  (junction 102) -> (junction 100) [order 1] : [SOC>0.0687&&SOC<0.1177]
  (junction 100) -> (junction 74) : {G=20.522/1000;}
  (junction 102) -> (junction 89) [order 2]
  (junction 89) -> (junction 94) [order 1] : [SOC>0.0197&&SOC<0.0687]
  (junction 94) -> (junction 96) : {G=100/1000;}
  (junction 89) -> (junction 99) [order 2]
  (junction 99) -> (junction 93) [order 1] : [SOC>0.0&&SOC<0.0197]
  (junction 93) -> (junction 90) : {G=100/1000;}
  (junction 99) -> (junction 105) [order 2]
  (junction 105) -> (junction 110)
  (junction 110) -> (junction 107) : {G=1;}
  data: SOC input; G output size=1

== matlab function PSOmodel/EKF/P_cov clac ==
  data: A input; P_Cov output; StaNoise input; P input
function P_Cov = CovMat(A, StaNoise, P)
A1 = [A(1) 0 0;0 A(2) 0;0 0 A(3)];
Qs = StaNoise(1);
Q1 = StaNoise(2);
Q2 = StaNoise(3);
P1 = [P(1) P(2) P(3); P(4) P(5) P(6); P(7) P(8) P(9)];
P2 = A1*P1*A1' + [Qs 0 0;0 Q1 0;0 0 Q2];  % 协方差矩阵预测
P_Cov = [P2(1,1) P2(1,2) P2(1,3) P2(2,1) P2(2,2) P2(2,3) P2(3,1) P2(3,2) P2(3,3)];

== matlab function PSOmodel/EKF/update P_cov ==
  data: P_Cov input; P_upd output size=[1 9]; K input; C input
function P_upd = CovUpd(P_Cov, K, C)
C = [C(1) C(2) C(3)];
P = [P_Cov(1) P_Cov(2)  P_Cov(3); P_Cov(4) P_Cov(5) P_Cov(6);P_Cov(7) P_Cov(8) P_Cov(9)];
P1 = P - K * C * P;   % 协方差矩阵更新
P_upd = [P1(1,1) P1(1,2) P1(1,3) P1(2,1) P1(2,2) P1(2,3) P1(3,1) P1(3,2) P1(3,3)];

== matlab function PSOmodel/EKF/calc K ==
  data: G input; P_Cov input; K output; R input; C input
function K = KalmanGain(G,P_Cov, R, C)
C1 = [C(1) C(2) C(3)];
P = [P_Cov(1) P_Cov(2)  P_Cov(3); P_Cov(4) P_Cov(5) P_Cov(6);P_Cov(7) P_Cov(8) P_Cov(9)];
K = G*P*C1'* (C1*P*C1'+R)^(-1);  % 增益

== stateflow chart PSOmodel/EKF/1_Chart ==
  (default) -> (junction 2)
  (junction 2) -> (junction 4) [order 1] : [SOC>0.6791&&SOC<0.7249]
  (junction 4) -> (junction 22) : {G=32.0857/100/2;}
  (junction 2) -> (junction 5) [order 2]
  (junction 5) -> (junction 6) [order 1] : [SOC>0.6332&&SOC<0.6791]
  (junction 6) -> (junction 28) : {G=12.245/100/2;}
  (junction 5) -> (junction 18) [order 2]
  (junction 18) -> (junction 19) [order 1] : [SOC>0.5874&&SOC<0.6332]
  (junction 19) -> (junction 30) : {G=12.7373/100/2;}
  (junction 18) -> (junction 35) [order 2]
  (junction 35) -> (junction 36) [order 1] : [SOC>0.5416&&SOC<0.5874]
  (junction 36) -> (junction 40) : {G=89.9935/100/2;}
  (junction 35) -> (junction 43) [order 2]
  (junction 43) -> (junction 41) [order 1] : [SOC>0.4957&&SOC<0.5416]
  (junction 41) -> (junction 32) : {G=61.4065/100/2;}
  (junction 43) -> (junction 50) [order 2]
  (junction 50) -> (junction 47) [order 1] : [SOC>0.4499&&SOC<0.4957]
  (junction 47) -> (junction 56) : {G=57.0579/100;}
  (junction 50) -> (junction 48) [order 2]
  (junction 48) -> (junction 51) [order 1] : [SOC>0.4040&&SOC<0.4499]
  (junction 51) -> (junction 55) : {G=62.6623/100;}
  (junction 48) -> (junction 72) [order 2]
  (junction 72) -> (junction 70) [order 1] : [SOC>0.3582&&SOC<0.4040]
  (junction 70) -> (junction 44) : {G=67.6477/100/2;}
  (junction 72) -> (junction 59) [order 2]
  (junction 59) -> (junction 64) [order 1] : [SOC>0.3123&&SOC<0.3582]
  (junction 64) -> (junction 66) : {G=66.2974/100/2;}
  (junction 59) -> (junction 69) [order 2]
  (junction 69) -> (junction 63) [order 1] : [SOC>0.2665&&SOC<0.3123]
  (junction 63) -> (junction 60) : {G=57.2898/100/2;}
  (junction 69) -> (junction 80) [order 2]
  (junction 80) -> (junction 77) [order 1] : [SOC>0.2207&&SOC<0.2665]
  (junction 77) -> (junction 86) : {G=46.9361/100/2;}
  (junction 80) -> (junction 78) [order 2]
  (junction 78) -> (junction 81) [order 1] : [SOC>0.1748&&SOC<0.2207]
  (junction 81) -> (junction 85) : {G=34.8887/100/2;}
  (junction 78) -> (junction 102) [order 2]
  (junction 102) -> (junction 100) [order 1] : [SOC>0.1290&&SOC<0.1748]
  (junction 100) -> (junction 74) : {G=25/100/2;}
  (junction 102) -> (junction 89) [order 2]
  (junction 89) -> (junction 94) [order 1] : [SOC>0.0831&&SOC<0.1290]
  (junction 94) -> (junction 96) : {G=21.0577/100/2;}
  (junction 89) -> (junction 99) [order 2]
  (junction 99) -> (junction 93) [order 1] : [SOC>0.0373&&SOC<0.0831]
  (junction 93) -> (junction 90) : {G=17.5/100/2;}
  (junction 99) -> (junction 105) [order 2]
  (junction 105) -> (junction 110)
  (junction 110) -> (junction 107) : {G=1;}
  data: SOC input; G output size=1

== stateflow chart PSOmodel/EKF/3_Chart ==
  (default) -> (junction 2)
  (junction 2) -> (junction 4) [order 1] : [SOC>0.6782&&SOC<0.7242]
  (junction 4) -> (junction 22) : {G=39.49/100;}
  (junction 2) -> (junction 5) [order 2]
  (junction 5) -> (junction 6) [order 1] : [SOC>0.6323&&SOC<0.6782]
  (junction 6) -> (junction 28) : {G=66.442/100;}
  (junction 5) -> (junction 18) [order 2]
  (junction 18) -> (junction 19) [order 1] : [SOC>0.5863&&SOC<0.6323]
  (junction 19) -> (junction 30) : {G=46.693/100;}
  (junction 18) -> (junction 35) [order 2]
  (junction 35) -> (junction 36) [order 1] : [SOC>0.5404&&SOC<0.5863]
  (junction 36) -> (junction 40) : {G=42.012/1000;}
  (junction 35) -> (junction 43) [order 2]
  (junction 43) -> (junction 41) [order 1] : [SOC>0.4944&&SOC<0.5404]
  (junction 41) -> (junction 32) : {G=48.935 /1000;}
  (junction 43) -> (junction 50) [order 2]
  (junction 50) -> (junction 47) [order 1] : [SOC>0.4484&&SOC<0.4944]
  (junction 47) -> (junction 56) : {G=58.346/1000;}
  (junction 50) -> (junction 48) [order 2]
  (junction 48) -> (junction 51) [order 1] : [SOC>0.4025&&SOC<0.4484]
  (junction 51) -> (junction 55) : {G=68.337/1000;}
  (junction 48) -> (junction 72) [order 2]
  (junction 72) -> (junction 70) [order 1] : [SOC>0.3565&&SOC<0.4025]
  (junction 70) -> (junction 44) : {G=72.2/1000;}
  (junction 72) -> (junction 59) [order 2]
  (junction 59) -> (junction 64) [order 1] : [SOC>0.3105&&SOC<0.3565]
  (junction 64) -> (junction 66) : {G=71.733/1000;}
  (junction 59) -> (junction 69) [order 2]
  (junction 69) -> (junction 63) [order 1] : [SOC>0.2646&&SOC<0.3105]
  (junction 63) -> (junction 60) : {G=66.624/1000;}
  (junction 69) -> (junction 80) [order 2]
  (junction 80) -> (junction 77) [order 1] : [SOC>0.2186&&SOC<0.2646]
  (junction 77) -> (junction 86) : {G=57.344/1000;}
  (junction 80) -> (junction 78) [order 2]
  (junction 78) -> (junction 81) [order 1] : [SOC>0.1726&&SOC<0.2186]
  (junction 81) -> (junction 85) : {G=47.041/1000;}
  (junction 78) -> (junction 102) [order 2]
  (junction 102) -> (junction 100) [order 1] : [SOC>0.1267&&SOC<0.1726]
  (junction 100) -> (junction 74) : {G=42.707/1000;}
  (junction 102) -> (junction 89) [order 2]
  (junction 89) -> (junction 94) [order 1] : [SOC>0.0807&&SOC<0.1267]
  (junction 94) -> (junction 96) : {G=38.886/1000;}
  (junction 89) -> (junction 99) [order 2]
  (junction 99) -> (junction 93) [order 1] : [SOC>0.0347&&SOC<0.0807]
  (junction 93) -> (junction 90) : {G=0/1000;}
  (junction 99) -> (junction 105) [order 2]
  (junction 105) -> (junction 110)
  (junction 110) -> (junction 107) : {G=1;}
  data: SOC input; G output size=1

== stateflow chart PSOmodel/EKF/Chart ==
  (default) -> (junction 2)
  (junction 2) -> (junction 4) [order 1] : [SOC>0.05&&SOC<0.95]
  (junction 2) -> (junction 5) [order 2] : {G=1;}
  (junction 4) -> (junction 6) : {G=G_in;}
  (junction 6) -> (junction 5)
  data: SOC input; G output size=1; G_in input size=1
